simulink model "MAVMODEL8S"  (R2020b)
settings: Solver=VariableStepAuto  StartTime=0.0  StopTime=30.0  RelTol=1e-3
values from neighbouring files (symbols this model uses):
  A = zeros(8)    [MAVLQG.m]
  B = zeros(8,4)    [MAVLQG.m]
  cMi = pinv(cM)    [MAVLQG.m]
  g = 9.81    [MAVLQG.m]
  k = 1.8409e-4    (= 0.00018409)    [MAVLQG.m]
  M = 1.280    (= 1.28)    [MAVLQG.m]
  x = [0 0 0  0 0  0 0 0]    [MAVLQG.m]
  zf = 0.5    [MAVLQG.m]
undefined symbols (not defined in the file or in its folder): Kd
settings Model: Creator=HENRY ODOEMELEM  LastModifiedBy=HENRY ODOEMELEM

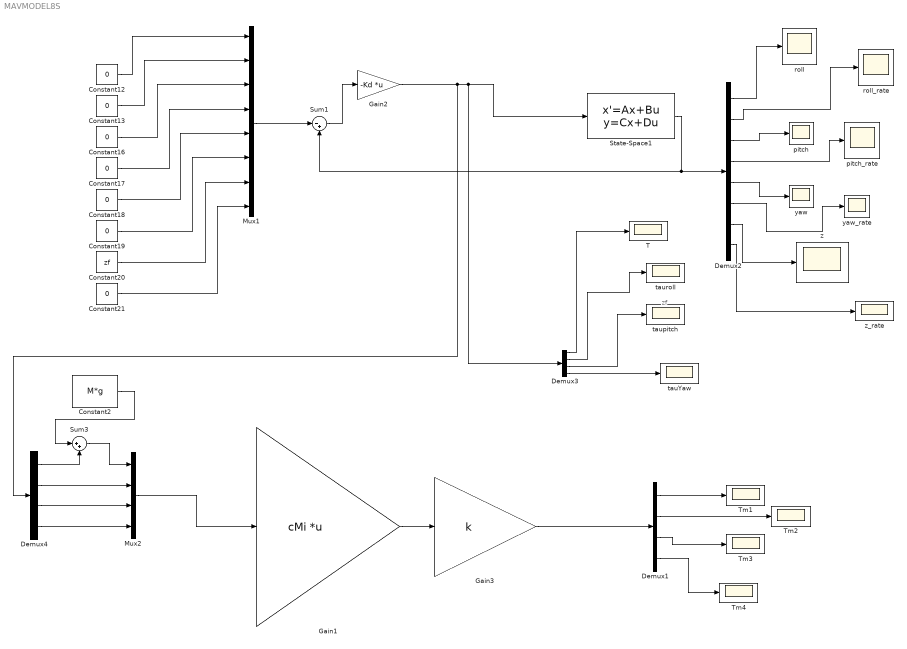
== system MAVMODEL8S ==
  note: zf
  Constant{12..13,16..19,21} (7 alike) : Constant  Value=0
  Constant2 : Constant  Value=M*g
  Constant20 : Constant  Value=zf
  Demux1 : Demux
  Demux2 : Demux  Outputs=8
  Demux3 : Demux
  Demux4 : Demux
  Gain1 : Gain  Gain=cMi  Multiplication=Matrix(K*u)
  Gain2 : Gain  Gain=-Kd  Multiplication=Matrix(K*u)
  Gain3 : Gain  Gain=k
  Mux1 : Mux  Inputs=8
  Mux2 : Mux
  State-Space1 : StateSpace  A=A  B=B  C=eye(8)  D=zeros(8,4)  InitialCondition=x  AbsoluteTolerance=0.00000000000000001
  Sum1 : Sum  Inputs=|-+
  Sum3 : Sum  Inputs=|++
  T : Scope
  Tm{1..4} (4 alike) : Scope
  pitch : Scope
  pitch_rate : Scope
  roll : Scope
  roll_rate : Scope
  tauYaw : Scope
  taupitch : Scope
  tauroll : Scope
  yaw : Scope
  yaw_rate : Scope
  z : Scope
  z_rate : Scope
  wires:
  Demux2/1 -> roll/1
  Mux1/1 -> Sum1/1
  Demux2/6 -> yaw_rate/1
  Constant21/1 -> Mux1/8
  Constant18/1 -> Mux1/5
  Constant16/1 -> Mux1/3
  Constant17/1 -> Mux1/4
  Demux2/7 -> z/1
  Constant13/1 -> Mux1/2
  Constant12/1 -> Mux1/1
  Constant20/1 -> Mux1/7
  Demux3/3 -> taupitch/1
  State-Space1/1 -> Demux2/1, Sum1/2
  Demux3/1 -> T/1
  Demux2/3 -> pitch/1
  Constant19/1 -> Mux1/6
  Sum1/1 -> Gain2/1
  Demux3/4 -> tauYaw/1
  Demux3/2 -> tauroll/1
  Demux2/5 -> yaw/1
  Demux2/2 -> roll_rate/1
  Demux2/8 -> z_rate/1
  Demux2/4 -> pitch_rate/1
  Demux1/1 -> Tm1/1
  Gain1/1 -> Gain3/1
  Demux1/2 -> Tm2/1
  Demux1/3 -> Tm3/1
  Demux1/4 -> Tm4/1
  Mux2/1 -> Gain1/1
  Demux4/3 -> Mux2/3
  Demux4/1 -> Sum3/2
  Sum3/1 -> Mux2/1
  Demux4/2 -> Mux2/2
  Constant2/1 -> Sum3/1
  Demux4/4 -> Mux2/4
  Gain2/1 -> Demux4/1, Demux3/1, State-Space1/1
  Gain3/1 -> Demux1/1
